simulink library "thermochemical"  (R2017b)
settings: Solver=VariableStepAuto  StartTime=0.0  StopTime=10.0  RelTol=1e-3
values from neighbouring files (symbols this model uses):
  c = conversion_factors()    [blk_clausius_clapeyron.m]    (also in blk_clausius_clapeyron_no_popup.m; blk_cold_room_closed_dry_air.m; blk_reactor_BaCl2_NH3_no_walls.m; blk_reactor_BaCl2_NH3_no_walls_state_space.m)
  cp = metal.cp    [blk_wall_simple.m]    (also in get_metal_properties.m = 390)
  fluid = get_param(blk,'fluid')    [blk_thermodynamic_properties_nonsaturated.m]    (also in blk_thermodynamic_properties_nonsaturated_interpreted.m; blk_thermodynamic_properties_saturated.m; blk_thermodynamic_properties_saturated_interpreted.m; blk_thermodynamic_properties_saturated_mix.m)
  gas = get_material_properties(x.gasName)    [blk_reactor_BaCl2_NH3_cylindrical_no_walls_fun1.m]
  h = get_param(gcb,'ObjectParameters')    [get_param_eval.m]
  rho = metal.rho    [blk_wall_simple.m]    (also in get_metal_properties.m = 8940)
  s = solve(eq,dx,'ReturnConditions',true)    [LMTD_inv.m]    (also in blk_wall_simple.m = get_param_eval(blk,'s'))
  u_gas_at_T_ref = -R * T_ref    [blk_reactor_BaCl2_NH3_no_walls.m]    (also in blk_reactor_BaCl2_NH3_no_walls_state_space.m)
undefined symbols (not defined in the file or in its folder): b_motor, BaCl2, beta, CoolProp, cP_binder, cP_gas, cP_s0, cv, dh_r_0, ENG, heat_exchanger_epsilonNTU_inv_simulink, heat_exchanger_epsilonNTU_simulink, J_motor, K_cin, kappa, Km_motor, La_motor, lookup2D_BreakPoint2, M_binder, N_binder, N_gas_free_volume_init, N_salt, NH3, nh3_v3, nu, P, phase, PID_D_motor, PID_I_motor, PID_P_motor, Ra_motor, Reactor_phase, T, T1, T2, T_init, Tr_init, Tr_ref, U_binder_at_Tr_ref, U_salt_at_X0_Tr_ref, Ur_init, V_void, Valve_regime, Vmax_motor, w_init_motor, X_init
libraries: thermochemical x247, simulink x54, dspsigops x3
(part 9 of 12)

== system thermochemical/Valves/Valve, gas, IEC 60534-2-1:2012 (exact)/Flow computation for compressible fluids, IEC 60534-2-1:2012/Valve regime ==
  In1 : Inport
  In2 : Inport  Port=2
  Enumerated Constant : simulink/Sources/Enumerated Constant  OutDataTypeStr=Enum: Valve_regime  Value=Valve_regime.Open_NonChocked  SampleTime=inf
      settings: SourceProductName=Simulink
  Enumerated Constant1 : simulink/Sources/Enumerated Constant  OutDataTypeStr=Enum: Valve_regime  Value=Valve_regime.Open_Chocked  SampleTime=inf
      settings: SourceProductName=Simulink
  Enumerated Constant2 : simulink/Sources/Enumerated Constant  OutDataTypeStr=Enum: Valve_regime  Value=Valve_regime.Closed  SampleTime=inf
      settings: SourceProductName=Simulink
  Switch1 : Switch  Criteria=u2 > Threshold
  Switch2 : Switch  Criteria=u2 > Threshold  Threshold=1e-5
  Out1 : Outport
  wires:
  In1/1 -> Switch2/2  "valve is closed"
  In2/1 -> Switch1/2  "non-chocked"
  Switch2/1 -> Out1/1  "regime"
  Enumerated Constant2/1 -> Switch2/3  "closed"
  Enumerated Constant1/1 -> Switch1/3  "chocked"
  Enumerated Constant/1 -> Switch1/1  "non-chocked"
  Switch1/1 -> Switch2/1

== system thermochemical/Valves/Valve, gas, IEC 60534-2-1:2012 (modified ideal gas approx.)/Glow computation for compressible fluids, IEC 60534-2-1:2012 (modified ideal gas assumption)/Subsystem ==
  P downstream (bar) : Inport
  P upstream (bar) : Inport  Port=2
  P upstream (bar)1 : Inport  Port=3
  Display{1..5} (5 alike) : Display
  Divide : Product  Inputs=*/
  Divide2 : Product  Inputs=*/
  Gain2 : Gain  Gain=xT
  "Heat capacity ratio of air @ (60°F, 1atm)" : Constant  Value=1.40
  Sign : Signum
  Sum3 : Sum  Inputs=-+
  Sum4 : Sum  Inputs=-+
  Switch1 : Switch  Criteria=u2 > Threshold
  non-chocked : Outport
  non-chocked2 : Outport  Port=2
  non-chocked1 : Outport  Port=3
  wires:
  Divide/1 -> Gain2/1, Display1/1  "Fgamma"
  "Heat capacity ratio of air @ (60°F, 1atm)"/1 -> Divide/2  "gamma air"
  P upstream (bar)1/1 -> Divide/1  "gamma upstream"
  Divide2/1 -> Switch1/1, Sum4/1, Display3/1  "x"
  Sum3/1 -> Divide2/1  "dP"
  Sum4/1 -> Sign/1
  Gain2/1 -> Sum4/2, non-chocked1/1, Display2/1, Switch1/3  "x chocked"
  Sign/1 -> non-chocked/1, Display4/1, Switch1/2  "non-chocked"
  P downstream (bar)/1 -> Sum3/1  "P downstream (bar)"
  P upstream (bar)/1 -> Sum3/2, Divide2/2  "P upstream (bar)"
  Switch1/1 -> non-chocked2/1, Display5/1  "x sizing"

== system thermochemical/Valves/Valve, gas, IEC 60534-2-1:2012 (modified ideal gas approx.)/Glow computation for compressible fluids, IEC 60534-2-1:2012 (modified ideal gas assumption)/Subsystem1 ==
  In1 : Inport
  In2 : Inport  Port=2
  Constant : Constant
  Display4 : Display
  Divide : Product  Inputs=*/
  Gain : Gain  Gain=3
  Sum3 : Sum  Inputs=+-|
  Y : Outport
  wires:
  Constant/1 -> Sum3/1
  In1/1 -> Divide/1  "x sizing"
  Gain/1 -> Divide/2
  Sum3/1 -> Y/1, Display4/1  "Y"
  In2/1 -> Gain/1  "x chocked"
  Divide/1 -> Sum3/2

== system thermochemical/Valves/Valve, gas, IEC 60534-2-1:2012 (modified ideal gas approx.)/Glow computation for compressible fluids, IEC 60534-2-1:2012 (modified ideal gas assumption)/Valve regime ==
  In1 : Inport
  In2 : Inport  Port=2
  Enumerated Constant : simulink/Sources/Enumerated Constant  OutDataTypeStr=Enum: Valve_regime  Value=Valve_regime.Open_NonChocked  SampleTime=inf
      settings: SourceProductName=Simulink
  Enumerated Constant1 : simulink/Sources/Enumerated Constant  OutDataTypeStr=Enum: Valve_regime  Value=Valve_regime.Open_Chocked  SampleTime=inf
      settings: SourceProductName=Simulink
  Enumerated Constant2 : simulink/Sources/Enumerated Constant  OutDataTypeStr=Enum: Valve_regime  Value=Valve_regime.Closed  SampleTime=inf
      settings: SourceProductName=Simulink
  Switch1 : Switch  Criteria=u2 > Threshold
  Switch2 : Switch  Criteria=u2 > Threshold  Threshold=1e-5
  Out1 : Outport
  wires:
  Switch1/1 -> Switch2/1
  Enumerated Constant/1 -> Switch1/1  "non-chocked"
  Enumerated Constant1/1 -> Switch1/3  "chocked"
  Enumerated Constant2/1 -> Switch2/3  "closed"
  Switch2/1 -> Out1/1  "regime"
  In2/1 -> Switch1/2  "non-chocked"
  In1/1 -> Switch2/2  "valve is closed"

== system thermochemical/Valves/Valve, gas, Swagelok model/Gas flow computation ('Swagelok' equations)/Sub-critical (P2 > 1//2 P1) ==
  note: In Matlab script notation:
  note: Reference:
      | Swagelok—TM Swagelok Company
      | © 1994, 1995, 2000, 2002 Swagelok Company
      | December 2007, R4
      | MS-06-84-E
  note: Flow Calculation (in SCFH),
      | sub-critical flow (gas at speed less than the speed of sound)
      | according to 'Swagelok' documentation
  note: % Sub-critical:
      | N2 = 22.67;
      | c = N2 * Pin_psi * (1-2/3*dP_psi/Pin_psi) * sqrt(dP_psi / (Pin_psi*Ggas*Tin_R));
      | SCFM = Cv * c;
      | SCFH = SCFM * 60;
  Ggas : Inport
  Ggas1 : Inport  Port=2
  T1 (°R) : Inport  Port=3
  P1 : Inport  Port=4
  dP : Inport  Port=5
  Constant : Constant
  Divide1 : Product  Inputs=**
  Divide3 : Product  Inputs=/*
  Divide4 : Product  Inputs=/*
  Divide5 : Product  Inputs=***
  Gain5 : Gain  Gain=2/3
  N2 : Gain  Gain=22.67
  Product1 : Product  Inputs=3
  SCFM to SCFH : Gain  Gain=60
  Sqrt : Sqrt  SaturateOnIntegerOverflow=on
  Sum3 : Sum  Inputs=+-|
  c : Outport
  wires:
  dP/1 -> Divide3/2, Divide4/2  "dP (psi)"
  Constant/1 -> Sum3/1
  Ggas/1 -> Product1/1  "Ggas"
  Divide3/1 -> Gain5/1  "dP/P1"
  Gain5/1 -> Sum3/2
  Sqrt/1 -> Divide5/1
  Sum3/1 -> Divide5/3  "1 - 2/3 dP/P1"
  T1 (°R)/1 -> Product1/2  "T1 (°R)"
  Divide5/1 -> N2/1
  Divide4/1 -> Sqrt/1
  N2/1 -> Divide1/2
  Product1/1 -> Divide4/1  "Ggas * T1 * P1"
  P1/1 -> Divide5/2, Product1/3, Divide3/1  "P1 (psi)"
  Ggas1/1 -> Divide1/1  "Cv"
  Divide1/1 -> SCFM to SCFH/1  "SCFM"
  SCFM to SCFH/1 -> c/1  "SCFH"

== system thermochemical/Valves/Valve, gas, Swagelok model/Gas flow computation ('Swagelok' equations)/Super-critical (P2 < 1//2 P1) ==
  note: % Super-critical:
      | N2 = 22.67;
      | c = 0.471 * N2 * Pin_psi * sqrt(1/(Ggas*Tin_R));
      | SCFM = Cv * c;
      | SCFH = SCFM * 60;
  note: Reference:
      | Swagelok—TM Swagelok Company
      | © 1994, 1995, 2000, 2002 Swagelok Company
      | December 2007, R4
      | MS-06-84-E
  note: In Matlab script notation:
  note: Flow Calculation (in SCFH),
      | super-critical (a.k.a. chocked) flow (gas at speed of sound)
      | according to 'Swagelok' documentation
  Ggas : Inport
  Ggas1 : Inport  Port=2
  T1 (°R) : Inport  Port=3
  P1 : Inport  Port=4
  Divide1 : Product  Inputs=**
  Divide5 : Product  Inputs=/*
  N1 : Gain  Gain=0.471
  N2 : Gain  Gain=22.67
  Product1 : Product
  SCFM to SCFH : Gain  Gain=60
  Sqrt : Sqrt  SaturateOnIntegerOverflow=on
  c : Outport
  wires:
  SCFM to SCFH/1 -> c/1  "SCFH"
  Divide1/1 -> SCFM to SCFH/1  "SCFM"
  Ggas1/1 -> Divide1/1  "Cv"
  P1/1 -> Divide5/2  "P1 (psi)"
  Product1/1 -> Sqrt/1  "Ggas * T1"
  N2/1 -> Divide1/2
  Divide5/1 -> N1/1
  T1 (°R)/1 -> Product1/2  "T1 (°R)"
  Sqrt/1 -> Divide5/1
  Ggas/1 -> Product1/1  "Ggas"
  N1/1 -> N2/1

== system thermochemical/Valves/Valve, gas, Swagelok model/Gas flow computation ('Swagelok' equations)/Valve regime ==
  In2 : Inport
  In1 : Inport  Port=2
  Enumerated Constant : simulink/Sources/Enumerated Constant  OutDataTypeStr=Enum: Valve_regime  Value=Valve_regime.Open_NonChocked  SampleTime=inf
      settings: SourceProductName=Simulink
  Enumerated Constant1 : simulink/Sources/Enumerated Constant  OutDataTypeStr=Enum: Valve_regime  Value=Valve_regime.Open_Chocked  SampleTime=inf
      settings: SourceProductName=Simulink
  Enumerated Constant2 : simulink/Sources/Enumerated Constant  OutDataTypeStr=Enum: Valve_regime  Value=Valve_regime.Closed  SampleTime=inf
      settings: SourceProductName=Simulink
  Switch1 : Switch  Criteria=u2 > Threshold
  Switch2 : Switch  Criteria=u2 > Threshold  Threshold=1e-5
  Out1 : Outport
  wires:
  In1/1 -> Switch2/2  "valve is closed"
  In2/1 -> Switch1/2  "P2 - 1/2 P1"
  Switch2/1 -> Out1/1  "regime"
  Enumerated Constant2/1 -> Switch2/3
  Enumerated Constant1/1 -> Switch1/3  "super-critical"
  Enumerated Constant/1 -> Switch1/1  "sub-critical"
  Switch1/1 -> Switch2/1

== system thermochemical/Valves/Valve, liquid (chocked condition not implemented)/Volume flow computation/Turbulent & non-choked flow conditions ==
  note: In Matlab script notation:
  note: Reference:
      | ANSI/ISA-75.01.01 (IEC 60534-2-1 Mod)-2007, eq. 1
  note: Flow Calculation
  note: % GPM computation:
      | N1 = 1;
      | GPM = Cv * N1 * sqrt(dP_psia/SG);
  Ggas : Inport
  dP : Inport  Port=2
  Ggas1 : Inport  Port=3
  Divide1 : Product  Inputs=**
  Divide4 : Product  Inputs=/*
  N1 : Gain
  Sqrt : Sqrt  SaturateOnIntegerOverflow=on
  c : Outport
  wires:
  dP/1 -> Divide4/2  "dP (psi)"
  Ggas/1 -> Divide4/1  "G (dimensionless)"
  Sqrt/1 -> N1/1
  Divide4/1 -> Sqrt/1
  N1/1 -> Divide1/2
  Ggas1/1 -> Divide1/1  "Cv"
  Divide1/1 -> c/1  "US gpm"

== system thermochemical/Valves/Valve, liquid (chocked condition not implemented)/Volume flow computation/Valve regime ==
  In1 : Inport
  Enumerated Constant1 : simulink/Sources/Enumerated Constant  OutDataTypeStr=Enum: Valve_regime  Value=Valve_regime.Open_NonChocked  SampleTime=inf
      settings: SourceProductName=Simulink
  Enumerated Constant2 : simulink/Sources/Enumerated Constant  OutDataTypeStr=Enum: Valve_regime  Value=Valve_regime.Closed  SampleTime=inf
      settings: SourceProductName=Simulink
  Switch2 : Switch  Criteria=u2 > Threshold  Threshold=1e-5
  Out1 : Outport
  wires:
  In1/1 -> Switch2/2  "valve is closed"
  Switch2/1 -> Out1/1  "regime"
  Enumerated Constant2/1 -> Switch2/3
  Enumerated Constant1/1 -> Switch2/1

== system thermochemical/Valves/Valve, liquid, IEC 60534-2-1:2012/Flow computation for incompressible fluids, IEC 60534-2-1:2012/Valve regime ==
  In1 : Inport
  In2 : Inport  Port=2
  Enumerated Constant : simulink/Sources/Enumerated Constant  OutDataTypeStr=Enum: Valve_regime  Value=Valve_regime.Open_NonChocked  SampleTime=inf
      settings: SourceProductName=Simulink
  Enumerated Constant1 : simulink/Sources/Enumerated Constant  OutDataTypeStr=Enum: Valve_regime  Value=Valve_regime.Open_Chocked  SampleTime=inf
      settings: SourceProductName=Simulink
  Enumerated Constant2 : simulink/Sources/Enumerated Constant  OutDataTypeStr=Enum: Valve_regime  Value=Valve_regime.Closed  SampleTime=inf
      settings: SourceProductName=Simulink
  Switch1 : Switch  Criteria=u2 > Threshold
  Switch2 : Switch  Criteria=u2 > Threshold  Threshold=1e-5
  Out1 : Outport
  wires:
  Switch1/1 -> Switch2/1
  Enumerated Constant/1 -> Switch1/1  "non-chocked"
  Enumerated Constant1/1 -> Switch1/3  "chocked"
  Enumerated Constant2/1 -> Switch2/3  "closed"
  Switch2/1 -> Out1/1  "regime"
  In2/1 -> Switch1/2  "non-chocked"
  In1/1 -> Switch2/2  "valve is closed"

== system thermochemical/Valves/Valve, liquid, IEC 60534-2-1:2012/Flow computation for incompressible fluids, IEC 60534-2-1:2012/dP sizing computation ==
  P upstream (bar) : Inport
  P upstream (bar)3 : Inport  Port=2
  P upstream (bar)2 : Inport  Port=3
  P upstream (bar)1 : Inport  Port=4
  Display{1..2,4..5} (4 alike) : Display
  FL factor : Constant  Value=FL
  Sign : Signum
  Sum3 : Sum  Inputs=-+
  Sum4 : Sum  Inputs=|-+
  Switch1 : Switch  Criteria=u2 > Threshold
  dP chocked computation : Subsystem
  non-chocked : Outport
  non-chocked2 : Outport  Port=2
  wires:
  Sum4/1 -> Sign/1
  Sign/1 -> Display4/1, non-chocked/1, Switch1/2  "non-chocked"
  P upstream (bar)/1 -> dP chocked computation/1(P upstream (bar)1), Sum3/2  "P upstream (bar)"
  Switch1/1 -> non-chocked2/1, Display5/1  "dP sizing (bar)"
  P upstream (bar)3/1 -> Sum3/1  "P downstream (bar)"
  Sum3/1 -> Sum4/1, Switch1/1, Display1/1  "dP (bar)"
  dP chocked computation/1(dP chocked (bar)) -> Sum4/2, Switch1/3, Display2/1  "dP chocked (bar)"
  P upstream (bar)2/1 -> dP chocked computation/2(P upstream (bar)2)  "Pv: absolute vapor pressure  of liquid at T upstream (bar)"
  P upstream (bar)1/1 -> dP chocked computation/3(P upstream (bar)3)  "Pc: absolute thermodynamic  critical pressure (bar)"
  FL factor/1 -> dP chocked computation/4(P upstream (bar)4)  "FL factor"

== system thermochemical/Walls/Wall, tube with//without fins/Subsystem1/Subsystem2 ==
  Display{1..4} (4 alike) : Display
  Product2 : Product
  Subsystem : thermochemical/Walls/Wall, tube with//without fins/Subsystem3/Subsystem
      settings: SourceProductName=@ Thermochemical
  Subsystem1 : Subsystem
  Subsystem2 : Subsystem
  Subsystem3 : thermochemical/Walls/Wall, tube with//without fins/Subsystem3/Subsystem3
      settings: SourceProductName=@ Thermochemical
  Switch1 : Switch  Criteria=u2 ~= 0
  s1 : Constant  Value=L_m
  s15 : Constant  Value=pitch_fin_mm
  s18 : Constant  Value=OD_mm
  s19 : Constant  Value=thickness_fin_mm
  s2 : Constant  Value=L_m
  s20 : Constant  Value=height_fin_mm
  s3 : Constant  Value=OD_mm
  s4 : Constant  Value=e_mm
  s5 : Constant  Value=0
  Total tube effective finned area (m2) : Outport
  Inner area (m2) : Outport  Port=2
  wires:
  Switch1/1 -> Display2/1, Total tube effective finned area (m2)/1  "Total finned tube volume (m3)"
  s19/1 -> Subsystem2/2(In2)
  s18/1 -> Subsystem2/1(In1)
  s20/1 -> Subsystem2/3(In4)
  s3/1 -> Subsystem1/1(In1)
  s2/1 -> Subsystem1/3(In3)
  s4/1 -> Subsystem1/2(In2)
  Subsystem1/1(Inner area (m2)) -> Display3/1, Inner area (m2)/1  "Bare tube volume (m3)"
  Subsystem2/1(Inner area (m2)) -> Display4/1, Product2/1
  s1/1 -> Subsystem3/1
  s15/1 -> Subsystem3/2
  Subsystem3/1 -> Display1/1, Product2/2
  Product2/1 -> Switch1/1  "Total finned tube volume (m3)"
  Subsystem/1 -> Switch1/2
  s5/1 -> Switch1/3

== system thermochemical/Walls/Wall, tube with//without fins/Subsystem3/Subsystem ==
  note: Check if any of the fin's parameters is zero
      | (in which case a 'bare tube' is considered)
  Compare To Constant : simulink/Logic and Bit Operations/Compare To Constant  relop=~=  const=0  OutDataTypeStr=boolean
  Mux : Mux  Inputs=3
  Product of Elements : Product  Inputs=*
  s1 : Constant  Value=thickness_fin_mm
  s4 : Constant  Value=pitch_fin_mm
  s5 : Constant  Value=height_fin_mm
  Out1 : Outport
  wires:
  Compare To Constant/1 -> Out1/1  "if == 1 : finned tube if == 0 : bare tube"
  s4/1 -> Mux/3
  s5/1 -> Mux/2
  Product of Elements/1 -> Compare To Constant/1
  s1/1 -> Mux/1
  Mux/1 -> Product of Elements/1

== system thermochemical/Walls/Wall, tube with//without fins/Subsystem3/Subsystem1 ==
  In1 : Inport
  In2 : Inport  Port=2
  In3 : Inport  Port=3
  Gain2 : Gain  Gain=1e-3
  Gain3 : Gain  Gain=1e-3
  Gain5 : Gain  Gain=1e-3
  Gain6 : Gain  Gain=pi
  Product4 : Product
  Sum2 : Sum  Inputs=+-
  Exposed tube area between two fins (m2) : Outport
  wires:
  Gain6/1 -> Product4/2
  Gain2/1 -> Sum2/2
  In2/1 -> Gain2/1  "thickness_fin_mm"
  Gain3/1 -> Gain6/1
  In3/1 -> Gain3/1  "OD_mm"
  In1/1 -> Gain5/1  "pitch_fin_mm"
  Gain5/1 -> Sum2/1
  Sum2/1 -> Product4/1  "Exposed length between two fins (m)"
  Product4/1 -> Exposed tube area between two fins (m2)/1  "Exposed tube area between two fins (m²)"

== system thermochemical/Walls/Wall, tube with//without fins/Subsystem3/Subsystem2 ==
  In1 : Inport
  In2 : Inport  Port=2
  In4 : Inport  Port=3
  Gain1 : Gain  Gain=pi/4
  Gain2 : Gain  Gain=2
  Gain3 : Gain  Gain=1e-3
  Gain4 : Gain  Gain=1e-3
  Gain5 : Gain  Gain=1e-3
  Gain6 : Gain  Gain=pi
  Math Function : Math  Operator=square  SaturateOnIntegerOverflow=on
  Math Function1 : Math  Operator=square  SaturateOnIntegerOverflow=on
  Product1 : Product
  Sum1 : Sum
  Sum2 : Sum  Inputs=+-
  Sum3 : Sum
  Inner area (m2) : Outport
  wires:
  Sum1/1 -> Inner area (m2)/1  "Area of  individual fin (m²)"
  Gain6/1 -> Sum1/2
  Product1/1 -> Gain6/1
  Gain3/1 -> Product1/2  "thickness_fin_m"
  In2/1 -> Gain3/1  "thickness_fin_mm"
  Gain2/1 -> Sum1/1
  Sum3/1 -> Math Function/1, Product1/1
  Gain1/1 -> Gain2/1  "Individual one-side  area of fin (m2)"
  In1/1 -> Gain5/1  "OD_mm"
  In4/1 -> Gain4/1  "height_fin_mm"
  Math Function/1 -> Sum2/1
  Math Function1/1 -> Sum2/2
  Sum2/1 -> Gain1/1
  Gain4/1 -> Sum3/1  "height_fin_m"
  Gain5/1 -> Sum3/2, Math Function1/1  "OD_m"

== system thermochemical/Walls/Wall, tube with//without fins/Subsystem3/Subsystem3 ==
  In1 : Inport
  In2 : Inport  Port=2
  Divide : Product  Inputs=*/
  Gain5 : Gain  Gain=1e-3
  Rounding Function : Rounding
  To avoid 'division by zero' error when pitch is zero : Saturate  UpperLimit=Inf  LowerLimit=1e-7
  Number of fins : Outport
  wires:
  To avoid 'division by zero' error when pitch is zero/1 -> Divide/2
  In2/1 -> Gain5/1  "pitch_fin_mm"
  Gain5/1 -> To avoid 'division by zero' error when pitch is zero/1
  Rounding Function/1 -> Number of fins/1  "Number of fins"
  Divide/1 -> Rounding Function/1
  In1/1 -> Divide/1  "L_m"

== system thermochemical/Walls/Wall, tube with//without fins/Subsystem3/Subsystem4 ==
  In1 : Inport
  In3 : Inport  Port=2
  Gain3 : Gain  Gain=1e-3
  Gain6 : Gain  Gain=pi
  Product4 : Product
  Exposed tube area between two fins (m2) : Outport
  wires:
  Gain6/1 -> Product4/2
  Gain3/1 -> Gain6/1
  Product4/1 -> Exposed tube area between two fins (m2)/1  "Bare tube  external area (m²)"
  In1/1 -> Product4/1  "L_m"
  In3/1 -> Gain3/1  "OD_mm"

== system thermochemical/Walls/Wall, tube with//without fins, with internal heat production/Subsystem1/Subsystem2 ==
  Display{1..4} (4 alike) : Display
  Product2 : Product
  Subsystem : thermochemical/Walls/Wall, tube with//without fins/Subsystem3/Subsystem
      settings: SourceProductName=@ Thermochemical
  Subsystem1 : Subsystem
  Subsystem2 : Subsystem
  Subsystem3 : thermochemical/Walls/Wall, tube with//without fins/Subsystem3/Subsystem3
      settings: SourceProductName=@ Thermochemical
  Switch1 : Switch  Criteria=u2 ~= 0
  s1 : Constant  Value=L_m
  s15 : Constant  Value=pitch_fin_mm
  s18 : Constant  Value=OD_mm
  s19 : Constant  Value=thickness_fin_mm
  s2 : Constant  Value=L_m
  s20 : Constant  Value=height_fin_mm
  s3 : Constant  Value=OD_mm
  s4 : Constant  Value=e_mm
  s5 : Constant  Value=0
  Total tube effective finned area (m2) : Outport
  Inner area (m2) : Outport  Port=2
  wires:
  s5/1 -> Switch1/3
  Subsystem/1 -> Switch1/2
  Product2/1 -> Switch1/1  "Total finned tube volume (m3)"
  Subsystem3/1 -> Product2/2, Display1/1
  s15/1 -> Subsystem3/2
  s1/1 -> Subsystem3/1
  Subsystem2/1(Inner area (m2)) -> Product2/1, Display4/1
  Subsystem1/1(Inner area (m2)) -> Inner area (m2)/1, Display3/1  "Bare tube volume (m3)"
  s4/1 -> Subsystem1/2(In2)
  s2/1 -> Subsystem1/3(In3)
  s3/1 -> Subsystem1/1(In1)
  s20/1 -> Subsystem2/3(In4)
  s18/1 -> Subsystem2/1(In1)
  s19/1 -> Subsystem2/2(In2)
  Switch1/1 -> Total tube effective finned area (m2)/1, Display2/1  "Total finned tube volume (m3)"

== system thermochemical/Walls/Wall, tube with//without fins, with internal heat production/Subsystem3/Subsystem ==
  note: Check if any of the fin's parameters is zero
      | (in which case a 'bare tube' is considered)
  Compare To Constant : simulink/Logic and Bit Operations/Compare To Constant  relop=~=  const=0  OutDataTypeStr=boolean
  Mux : Mux  Inputs=3
  Product of Elements : Product  Inputs=*
  s1 : Constant  Value=thickness_fin_mm
  s4 : Constant  Value=pitch_fin_mm
  s5 : Constant  Value=height_fin_mm
  Out1 : Outport
  wires:
  Mux/1 -> Product of Elements/1
  s1/1 -> Mux/1
  Product of Elements/1 -> Compare To Constant/1
  s5/1 -> Mux/2
  s4/1 -> Mux/3
  Compare To Constant/1 -> Out1/1  "if == 1 : finned tube if == 0 : bare tube"

== system thermochemical/Walls/Wall, tube with//without fins, with internal heat production/Subsystem3/Subsystem1 ==
  In1 : Inport
  In2 : Inport  Port=2
  In3 : Inport  Port=3
  Gain2 : Gain  Gain=1e-3
  Gain3 : Gain  Gain=1e-3
  Gain5 : Gain  Gain=1e-3
  Gain6 : Gain  Gain=pi
  Product4 : Product
  Sum2 : Sum  Inputs=+-
  Exposed tube area between two fins (m2) : Outport
  wires:
  Product4/1 -> Exposed tube area between two fins (m2)/1  "Exposed tube area between two fins (m²)"
  Sum2/1 -> Product4/1  "Exposed length between two fins (m)"
  Gain5/1 -> Sum2/1
  In1/1 -> Gain5/1  "pitch_fin_mm"
  In3/1 -> Gain3/1  "OD_mm"
  Gain3/1 -> Gain6/1
  In2/1 -> Gain2/1  "thickness_fin_mm"
  Gain2/1 -> Sum2/2
  Gain6/1 -> Product4/2

== system thermochemical/Walls/Wall, tube with//without fins, with internal heat production/Subsystem3/Subsystem2 ==
  In1 : Inport
  In2 : Inport  Port=2
  In4 : Inport  Port=3
  Gain1 : Gain  Gain=pi/4
  Gain2 : Gain  Gain=2
  Gain3 : Gain  Gain=1e-3
  Gain4 : Gain  Gain=1e-3
  Gain5 : Gain  Gain=1e-3
  Gain6 : Gain  Gain=pi
  Math Function : Math  Operator=square  SaturateOnIntegerOverflow=on
  Math Function1 : Math  Operator=square  SaturateOnIntegerOverflow=on
  Product1 : Product
  Sum1 : Sum
  Sum2 : Sum  Inputs=+-
  Sum3 : Sum
  Inner area (m2) : Outport
  wires:
  Gain5/1 -> Math Function1/1, Sum3/2  "OD_m"
  Gain4/1 -> Sum3/1  "height_fin_m"
  Sum2/1 -> Gain1/1
  Math Function1/1 -> Sum2/2
  Math Function/1 -> Sum2/1
  In4/1 -> Gain4/1  "height_fin_mm"
  In1/1 -> Gain5/1  "OD_mm"
  Gain1/1 -> Gain2/1  "Individual one-side  area of fin (m2)"
  Sum3/1 -> Product1/1, Math Function/1
  Gain2/1 -> Sum1/1
  In2/1 -> Gain3/1  "thickness_fin_mm"
  Gain3/1 -> Product1/2  "thickness_fin_m"
  Product1/1 -> Gain6/1
  Gain6/1 -> Sum1/2
  Sum1/1 -> Inner area (m2)/1  "Area of  individual fin (m²)"

== system thermochemical/Walls/Wall, tube with//without fins, with internal heat production/Subsystem3/Subsystem3 ==
  In1 : Inport
  In2 : Inport  Port=2
  Divide : Product  Inputs=*/
  Gain5 : Gain  Gain=1e-3
  Rounding Function : Rounding
  To avoid 'division by zero' error when pitch is zero : Saturate  UpperLimit=Inf  LowerLimit=1e-7
  Number of fins : Outport
  wires:
  In1/1 -> Divide/1  "L_m"
  Divide/1 -> Rounding Function/1
  Rounding Function/1 -> Number of fins/1  "Number of fins"
  Gain5/1 -> To avoid 'division by zero' error when pitch is zero/1
  In2/1 -> Gain5/1  "pitch_fin_mm"
  To avoid 'division by zero' error when pitch is zero/1 -> Divide/2

== system thermochemical/Walls/Wall, tube with//without fins, with internal heat production/Subsystem3/Subsystem4 ==
  In1 : Inport
  In3 : Inport  Port=2
  Gain3 : Gain  Gain=1e-3
  Gain6 : Gain  Gain=pi
  Product4 : Product
  Exposed tube area between two fins (m2) : Outport
  wires:
  In3/1 -> Gain3/1  "OD_mm"
  In1/1 -> Product4/1  "L_m"
  Product4/1 -> Exposed tube area between two fins (m2)/1  "Bare tube  external area (m²)"
  Gain3/1 -> Gain6/1
  Gain6/1 -> Product4/2

== system thermochemical/Control volumes/Two-phase saturated fluid control volume (without walls) (without algebraic loop)/Two-phase control volume state-space functions/f1/Subsystem ==
  In2 : Inport
  In3 : Inport  Port=2
  2 : Constant  Value=V
  3 : Constant  Value=V
  Derivative in the two-phase region ∂u/∂v|T : thermochemical/Thermodynamic fluid properties/Derivative in the two-phase region ∂u//∂v|T  fluid=fluid
      settings: SourceProductName=@ Thermochemical
  Product3 : Product  Inputs=**
  Product4 : Product  Inputs=*/
  Product5 : Product  Inputs=*/
  Sum1 : Sum  Inputs=+-
  Terminator : Terminator
  Thermodynamic property (saturated vapor-liquid mix) : thermochemical/Thermodynamic fluid properties/Thermodynamic property  (saturated vapor-liquid mix)  sel=u(T) (J/mol)  fluid=fluid  lookup1D_BreakPoint=0  lookup1D_Data1=fluid.sat.liq.u_molar  lookup1D_Data2=fluid.sat.vap.u_molar
      settings: SourceProductName=@ Thermochemical
  Vapor quality & Liquid volumetric fraction : thermochemical/Thermodynamic fluid properties/Vapor quality & Liquid  volumetric fraction  fluid=fluid
      settings: SourceProductName=@ Thermochemical
  Out1 : Outport
  wires:
  Product4/1 -> Sum1/2
  Sum1/1 -> Product3/1
  Derivative in the two-phase region ∂u/∂v|T/1 -> Sum1/1
  3/1 -> Vapor quality & Liquid volumetric fraction/3
  2/1 -> Product5/1
  Vapor quality & Liquid volumetric fraction/1 -> Thermodynamic property (saturated vapor-liquid mix)/2
  Product3/1 -> Out1/1  "∂U/∂v|T (J.mol/m³) (two-phase)"
  Product5/1 -> Product3/2, Vapor quality & Liquid volumetric fraction/2  "V/v = N (mol)"
  In3/1 -> Product4/2, Product5/2  "v (m3/mol)"
  In2/1 -> Derivative in the two-phase region ∂u/∂v|T/1, Thermodynamic property (saturated vapor-liquid mix)/1, Vapor quality & Liquid volumetric fraction/1  "T (K)"
  Thermodynamic property (saturated vapor-liquid mix)/1 -> Product4/1
  Vapor quality & Liquid volumetric fraction/2 -> Terminator/1

== system thermochemical/Control volumes/Two-phase saturated fluid control volume (without walls) (without algebraic loop)/Two-phase control volume state-space functions/f1/Subsystem1 ==
  In2 : Inport
  In3 : Inport  Port=2
  2 : Constant  Value=V
  3 : Constant  Value=V
  Derivative in the two-phase region ∂u/∂T|v : thermochemical/Thermodynamic fluid properties/Derivative in the two-phase region ∂u//∂T|v  fluid=fluid
      settings: SourceProductName=@ Thermochemical
  Product3 : Product  Inputs=**
  Product5 : Product  Inputs=*/
  Terminator : Terminator
  Vapor quality & Liquid volumetric fraction : thermochemical/Thermodynamic fluid properties/Vapor quality & Liquid  volumetric fraction  fluid=fluid
      settings: SourceProductName=@ Thermochemical
  Out1 : Outport
  wires:
  Vapor quality & Liquid volumetric fraction/2 -> Terminator/1
  In2/1 -> Derivative in the two-phase region ∂u/∂T|v/1, Vapor quality & Liquid volumetric fraction/1  "T (K)"
  In3/1 -> Product5/2  "v (m3/mol)"
  Product5/1 -> Product3/2, Vapor quality & Liquid volumetric fraction/2  "V/v = N (mol)"
  Product3/1 -> Out1/1  "∂U/∂T|v (J/K) (two-phase)"
  Vapor quality & Liquid volumetric fraction/1 -> Derivative in the two-phase region ∂u/∂T|v/2
  2/1 -> Product5/1
  3/1 -> Vapor quality & Liquid volumetric fraction/3
  Derivative in the two-phase region ∂u/∂T|v/1 -> Product3/1

== system thermochemical/Heat exchangers/Heat Exchanger, e-NTU method (UA input) Loop 2: water/Subsystem/Subsystem1/Average ==
  In1 : Inport
  In2 : Inport  Port=2
  Gain : Gain  Gain=0.5
  Sum : Sum
  Out1 : Outport
  wires:
  Gain/1 -> Out1/1  "avg"
  In1/1 -> Sum/1  "In 1"
  In2/1 -> Sum/2  "In 2"
  Sum/1 -> Gain/1

== system thermochemical/Heat exchangers/Heat Exchanger, e-NTU method (epsilon input) Loop 2: water/Subsystem/Subsystem1/Average ==
  In1 : Inport
  In2 : Inport  Port=2
  Gain : Gain  Gain=0.5
  Sum : Sum
  Out1 : Outport
  wires:
  Sum/1 -> Gain/1
  In2/1 -> Sum/2  "In 2"
  In1/1 -> Sum/1  "In 1"
  Gain/1 -> Out1/1  "avg"

== system thermochemical/Reactors/Reactor, BaCl2//NH3, state-space form, [Tr, Ng, X] as state variables, no algebraic loops, ideal gas in void volume, ideal gas in salt/Reactor, BaCl2//NH3, no walls, state-space form, [Tr, Ng, X] as state variables, no algebraic loops, ideal gas in void volume/Reactor, no walls, state space form/Reactor output function ==
  In1 : Inport
  Clausius-Clapeyron : thermochemical/Thermodynamic fluid properties/Clausius-Clapeyron  sel_1=P(T)  sel_2=BaCl2/NH3
      settings: SourceProductName=@ Thermochemical
  Demux : Demux  Outputs=3
  Enthalpy of ideal gas : thermochemical/Thermodynamic fluid properties/Enthalpy of ideal gas  T_ref=T_ref  cP_gas=cP_gas  h_gas_at_T_ref="u_gas_at_T_ref  + R * T_ref"
      settings: SourceProductName=@ Thermochemical
  Gain4 : Gain  Gain=nu*N_salt
  Gain7 : Gain  Gain=1/V_void
  Ideal gas equation of state : thermochemical/Thermodynamic fluid properties/Ideal gas equation of state  sel=P(T,rho)  R=8.3145  Pa_to_bar=1e-5  bar_to_Pa=1e5
      settings: SourceProductName=@ Thermochemical
  Mux : Mux
  Reactor phase : Subsystem
  Reactor's internal energy equation : thermochemical/Reactors/Reactor's internal energy equation  Tr_ref=T_ref  N_salt=N_salt  cP_s0=cP_s0  U_salt_at_X0_Tr_ref=U_salt_at_X0_T_ref  N_binder=N_binder  M_binder=M_binder  cP_binder=cP_binder  U_binder_at_Tr_ref=U_binder_at_T_ref  V_void=V_void  gas_model_void_volume=Ideal gas model  gas_model_salt=Ideal gas model  is_ideal_gas_in_void_volume=1  is_ideal_gas_in_salt=1  fluid=fluid  cP_gas=cP_gas  u_gas_at_Tr_ref=u_gas_at_T_ref  nu=nu  dh_r=dh_r_0  R=8.314472
      settings: SourceProductName=@ Thermochemical
  Sum16 : Sum  Inputs=+-|
  Sum4 : Sum  Inputs=|+-
  Terminator : Terminator
  Out1 : Outport
  Out2 : Outport  Port=2
  wires:
  Demux/3 -> Gain4/1, Mux/3, Reactor's internal energy equation/1  "x(3) = X (0..1)"
  Demux/1 -> Mux/1, Clausius-Clapeyron/1, Enthalpy of ideal gas/1, Ideal gas equation of state/1, Reactor's internal energy equation/3  "x(1) = T (K)"
  Reactor's internal energy equation/1 -> Terminator/1  "Ur (J)"
  Demux/2 -> Sum4/1  "x(2) = Ngas,total (mol)"
  Sum16/1 -> Reactor phase/1(In1)
  Clausius-Clapeyron/1 -> Sum16/2  "P eq (bar)"
  Reactor phase/1(Out1) -> Out2/1  "Reactor phase"
  Gain7/1 -> Ideal gas equation of state/2
  Enthalpy of ideal gas/1 -> Mux/4  "h gas free volume (J/mol)"
  Ideal gas equation of state/1 -> Mux/2, Sum16/1  "P (bar)"
  Sum4/1 -> Reactor's internal energy equation/2, Gain7/1  "Ngas,void"
  Gain4/1 -> Sum4/2
  Mux/1 -> Out1/1  "Y(vector)"
  In1/1 -> Demux/1  "X(vector)"

== system thermochemical/Reactors/Reactor, BaCl2//NH3, state-space form, [Tr, Ng, X] as state variables, no algebraic loops, ideal gas in void volume, ideal gas in salt/Reactor, BaCl2//NH3, no walls, state-space form, [Tr, Ng, X] as state variables, no algebraic loops, ideal gas in void volume/Reactor, no walls, state space form/Reactor state-space functions ==
  In1 : Inport
  In2 : Inport  Port=2
  Mux : Mux  Inputs=3
  f1 : Subsystem
  f2 : Subsystem
  f3 : Subsystem
  Out2 : Outport
  wires:
  In2/1 -> f1/2(In1), f3/2(In2), f2/2(In2)  "U(vector)"
  In1/1 -> f1/1(In6), f2/1(In6), f3/1(In6)  "X(vector)"
  Mux/1 -> Out2/1  "dX/dt(vector)"
  f1/1(Out2) -> Mux/1
  f3/1(Out2) -> Mux/3
  f2/1(Out2) -> Mux/2

== system thermochemical/Reactors/Reactor, BaCl2//NH3, state-space form, [Tr, Ng, X] as state variables, no algebraic loops, real gas in void volume, ideal gas in salt/Reactor, BaCl2//NH3, no walls, state-space form, [Tr, Ng, X] as state variables, no algebraic loops, real gas in void volume, ideal gas in salt/Reactor, no walls, state space form/Reactor output function ==
  In1 : Inport
  Clausius-Clapeyron : thermochemical/Thermodynamic fluid properties/Clausius-Clapeyron  sel_1=P(T)  sel_2=BaCl2/NH3
      settings: SourceProductName=@ Thermochemical
  Demux : Demux  Outputs=3
  Gain4 : Gain  Gain=nu*N_salt
  Gain7 : Gain  Gain=1/V_void
  Mux : Mux
  Reactor phase : Subsystem
  Reactor's internal energy equation : thermochemical/Reactors/Reactor's internal energy equation  Tr_ref=T_ref  N_salt=N_salt  cP_s0=cP_s0  U_salt_at_X0_Tr_ref=U_salt_at_X0_T_ref  N_binder=N_binder  M_binder=M_binder  cP_binder=cP_binder  U_binder_at_Tr_ref=U_binder_at_T_ref  V_void=V_void  gas_model_void_volume=Real gas model  gas_model_salt=Ideal gas model  is_ideal_gas_in_void_volume=-1  is_ideal_gas_in_salt=1  fluid=fluid  cP_gas=cP_gas  u_gas_at_Tr_ref=u_gas_at_T_ref  nu=nu  dh_r=dh_r_0  R=8.314472
      settings: SourceProductName=@ Thermochemical
  Sum16 : Sum  Inputs=+-|
  Sum4 : Sum  Inputs=|+-
  Terminator : Terminator
  Thermodynamic property (non-saturated) : thermochemical/Thermodynamic fluid properties/Thermodynamic  property (non-saturated)  sel=h(T,rho)  fluid=fluid  reciprocVar=-1  lookup2D_BreakPoint1=fluid.no_sat.T_rho_indep.var_indep.T  lookup2D_BreakPoint2=fluid.no_sat.T_rho_indep.var_indep.rho_molar  lookup2D_Data=fluid.no_sat.T_rho_indep.var_dep.h_molar
      settings: SourceProductName=@ Thermochemical
  Thermodynamic property (non-saturated)1 : thermochemical/Thermodynamic fluid properties/Thermodynamic  property (non-saturated)  sel=P(T,rho)  fluid=fluid  reciprocVar=-1  lookup2D_BreakPoint1=fluid.no_sat.T_rho_indep.var_indep.T  lookup2D_BreakPoint2=fluid.no_sat.T_rho_indep.var_indep.rho_molar  lookup2D_Data=fluid.no_sat.T_rho_indep.var_dep.P
      settings: SourceProductName=@ Thermochemical
  Out1 : Outport
  Out2 : Outport  Port=2
  wires:
  Reactor's internal energy equation/1 -> Terminator/1  "Ur (J)"
  In1/1 -> Demux/1  "X(vector)"
  Mux/1 -> Out1/1  "Y(vector)"
  Gain4/1 -> Sum4/2
  Sum4/1 -> Reactor's internal energy equation/2, Gain7/1  "Ngas,void"
  Thermodynamic property (non-saturated)1/1 -> Sum16/1, Mux/2  "P (bar)"
  Demux/3 -> Mux/3, Gain4/1, Reactor's internal energy equation/1  "X (0..1)"
  Thermodynamic property (non-saturated)/1 -> Mux/4  "h gas free volume (J/mol)"
  Demux/2 -> Sum4/1  "Ngas,total (mol)"
  Demux/1 -> Clausius-Clapeyron/1, Thermodynamic property (non-saturated)/1, Thermodynamic property (non-saturated)1/1, Mux/1, Reactor's internal energy equation/3  "T (K)"
  Gain7/1 -> Thermodynamic property (non-saturated)/2, Thermodynamic property (non-saturated)1/2
  Reactor phase/1(Out1) -> Out2/1  "Reactor phase"
  Clausius-Clapeyron/1 -> Sum16/2  "P eq (bar)"
  Sum16/1 -> Reactor phase/1(In1)

== system thermochemical/Reactors/Reactor, BaCl2//NH3, state-space form, [Tr, Ng, X] as state variables, no algebraic loops, real gas in void volume, ideal gas in salt/Reactor, BaCl2//NH3, no walls, state-space form, [Tr, Ng, X] as state variables, no algebraic loops, real gas in void volume, ideal gas in salt/Reactor, no walls, state space form/Reactor state-space functions ==
  In1 : Inport
  In2 : Inport  Port=2
  Mux : Mux  Inputs=3
  f1 : Subsystem
  f2 : Subsystem
  f3 : Subsystem
  Out2 : Outport
  wires:
  f2/1(Out2) -> Mux/2
  f3/1(Out2) -> Mux/3
  f1/1(Out2) -> Mux/1
  Mux/1 -> Out2/1  "dX/dt(vector)"
  In1/1 -> f3/1(In6), f2/1(In6), f1/1(In6)  "X(vector)"
  In2/1 -> f2/2(In2), f3/2(In2), f1/2(In1)  "U(vector)"

== system thermochemical/Reactors/Reactor, BaCl2//NH3, state-space form, [Tr, Ng, X] as state variables, no algebraic loops, real gas in void volume, real gas in salt/Reactor, BaCl2//NH3, no walls, state-space form, [Tr, Ng, X] as state variables, no algebraic loops, real gas in void volume, real gas in salt/Reactor, no walls, state space form/Reactor output function ==
  In1 : Inport
  Clausius-Clapeyron : thermochemical/Thermodynamic fluid properties/Clausius-Clapeyron  sel_1=P(T)  sel_2=BaCl2/NH3
      settings: SourceProductName=@ Thermochemical
  Demux : Demux  Outputs=3
  Gain4 : Gain  Gain=nu*N_salt
  Gain7 : Gain  Gain=1/V_void
  Mux : Mux
  Reactor phase : Subsystem
  Reactor's internal energy equation : thermochemical/Reactors/Reactor's internal energy equation  Tr_ref=T_ref  N_salt=N_salt  cP_s0=cP_s0  U_salt_at_X0_Tr_ref=U_salt_at_X0_T_ref  N_binder=N_binder  M_binder=M_binder  cP_binder=cP_binder  U_binder_at_Tr_ref=U_binder_at_T_ref  V_void=V_void  gas_model_void_volume=Real gas model  gas_model_salt=Real gas model  is_ideal_gas_in_void_volume=-1  is_ideal_gas_in_salt=-1  fluid=fluid  cP_gas=cP_gas  u_gas_at_Tr_ref=u_gas_at_T_ref  nu=nu  dh_r=dh_r_0  R=8.314472
      settings: SourceProductName=@ Thermochemical
  Sum16 : Sum  Inputs=+-|
  Sum4 : Sum  Inputs=|+-
  Terminator : Terminator
  Thermodynamic property (non-saturated) : thermochemical/Thermodynamic fluid properties/Thermodynamic  property (non-saturated)  sel=h(T,rho)  fluid=fluid  reciprocVar=-1  lookup2D_BreakPoint1=fluid.no_sat.T_rho_indep.var_indep.T  lookup2D_BreakPoint2=fluid.no_sat.T_rho_indep.var_indep.rho_molar  lookup2D_Data=fluid.no_sat.T_rho_indep.var_dep.h_molar
      settings: SourceProductName=@ Thermochemical
  Thermodynamic property (non-saturated)1 : thermochemical/Thermodynamic fluid properties/Thermodynamic  property (non-saturated)  sel=P(T,rho)  fluid=fluid  reciprocVar=-1  lookup2D_BreakPoint1=fluid.no_sat.T_rho_indep.var_indep.T  lookup2D_BreakPoint2=fluid.no_sat.T_rho_indep.var_indep.rho_molar  lookup2D_Data=fluid.no_sat.T_rho_indep.var_dep.P
      settings: SourceProductName=@ Thermochemical
  Out1 : Outport
  Out2 : Outport  Port=2
  wires:
  Sum16/1 -> Reactor phase/1(In1)
  Clausius-Clapeyron/1 -> Sum16/2  "P eq (bar)"
  Reactor phase/1(Out1) -> Out2/1  "Reactor phase"
  Gain7/1 -> Thermodynamic property (non-saturated)1/2, Thermodynamic property (non-saturated)/2
  Demux/1 -> Reactor's internal energy equation/3, Mux/1, Thermodynamic property (non-saturated)1/1, Thermodynamic property (non-saturated)/1, Clausius-Clapeyron/1  "T (K)"
  Demux/2 -> Sum4/1  "Ngas,total (mol)"
  Thermodynamic property (non-saturated)/1 -> Mux/4  "h gas free volume (J/mol)"
  Demux/3 -> Reactor's internal energy equation/1, Gain4/1, Mux/3  "X (0..1)"
  Thermodynamic property (non-saturated)1/1 -> Mux/2, Sum16/1  "P (bar)"
  Sum4/1 -> Reactor's internal energy equation/2, Gain7/1  "Ngas,void"
  Gain4/1 -> Sum4/2
  Mux/1 -> Out1/1  "Y(vector)"
  In1/1 -> Demux/1  "X(vector)"
  Reactor's internal energy equation/1 -> Terminator/1  "Ur (J)"

== system thermochemical/Reactors/Reactor, BaCl2//NH3, state-space form, [Tr, Ng, X] as state variables, no algebraic loops, real gas in void volume, real gas in salt/Reactor, BaCl2//NH3, no walls, state-space form, [Tr, Ng, X] as state variables, no algebraic loops, real gas in void volume, real gas in salt/Reactor, no walls, state space form/Reactor state-space functions ==
  In1 : Inport
  In2 : Inport  Port=2
  Mux : Mux  Inputs=3
  f1 : Subsystem
  f2 : Subsystem
  f3 : Subsystem
  Out2 : Outport
  wires:
  In2/1 -> f1/2(In1), f3/2(In2), f2/2(In2)  "U(vector)"
  In1/1 -> f1/1(In6), f2/1(In6), f3/1(In6)  "X(vector)"
  Mux/1 -> Out2/1  "dX/dt(vector)"
  f1/1(Out2) -> Mux/1
  f3/1(Out2) -> Mux/3
  f2/1(Out2) -> Mux/2

== system thermochemical/Reactors/Reactor, BaCl2//NH3, state-space form, [Ur, Ng, X] as state variables, no algebraic loops, ideal gas in void volume, ideal gas in salt/Reactor, BaCl2//NH3, no walls, state-space form, [Ur, Ng, X] as state variables, no algebraic loops, ideal gas in void volume, ideal gas in salt/Reactor, no walls, state space form/Initial conditions ==
  Gain1 : Gain  Gain=N_salt * nu
  Initial condition : Constant  Value=X_init
  Initial condition1 : Constant  Value=N_gas_free_volume_init
  Initial condition2 : Constant  Value=Tr_init
  Mux : Mux  Inputs=3
  Reactor's internal energy equation : thermochemical/Reactors/Reactor's internal energy equation  Tr_ref=T_ref  N_salt=N_salt  cP_s0=cP_s0  U_salt_at_X0_Tr_ref=U_salt_at_X0_T_ref  N_binder=N_binder  M_binder=M_binder  cP_binder=cP_binder  U_binder_at_Tr_ref=U_binder_at_T_ref  V_void=V_void  gas_model_void_volume=Ideal gas model  gas_model_salt=Ideal gas model  is_ideal_gas_in_void_volume=1  is_ideal_gas_in_salt=1  fluid=fluid  cP_gas=cP_gas  u_gas_at_Tr_ref=u_gas_at_T_ref  nu=nu  dh_r=dh_r_0  R=8.314472
      settings: SourceProductName=@ Thermochemical
  Sum4 : Sum  Inputs=++|
  Out2 : Outport
  wires:
  Mux/1 -> Out2/1  "X0 (vector)"
  Initial condition/1 -> Reactor's internal energy equation/1, Gain1/1, Mux/3  "x(3) = X (0..1)"
  Initial condition1/1 -> Reactor's internal energy equation/2, Sum4/1
  Reactor's internal energy equation/1 -> Mux/1  "x(1) = Ur (J)"
  Initial condition2/1 -> Reactor's internal energy equation/3
  Sum4/1 -> Mux/2  "x(2) = Ngas,total (mol)"
  Gain1/1 -> Sum4/2

== system thermochemical/Reactors/Reactor, BaCl2//NH3, state-space form, [Ur, Ng, X] as state variables, no algebraic loops, ideal gas in void volume, ideal gas in salt/Reactor, BaCl2//NH3, no walls, state-space form, [Ur, Ng, X] as state variables, no algebraic loops, ideal gas in void volume, ideal gas in salt/Reactor, no walls, state space form/Reactor output function ==
  In1 : Inport
  Clausius-Clapeyron : thermochemical/Thermodynamic fluid properties/Clausius-Clapeyron  sel_1=P(T)  sel_2=BaCl2/NH3
      settings: SourceProductName=@ Thermochemical
  Demux : Demux  Outputs=3
  Enthalpy of ideal gas : thermochemical/Thermodynamic fluid properties/Enthalpy of ideal gas  T_ref=T_ref  cP_gas=cP_gas  h_gas_at_T_ref="u_gas_at_T_ref  + R * T_ref"
      settings: SourceProductName=@ Thermochemical
  Gain4 : Gain  Gain=nu*N_salt
  Gain7 : Gain  Gain=1/V_void
  Ideal gas equation of state : thermochemical/Thermodynamic fluid properties/Ideal gas equation of state  sel=P(T,rho)  R=8.3145  Pa_to_bar=1e-5  bar_to_Pa=1e5
      settings: SourceProductName=@ Thermochemical
  Mux : Mux
  Reactor phase : Subsystem
  Sum16 : Sum  Inputs=+-|
  Sum4 : Sum  Inputs=|+-
  Tr = inv(g[X(vector)]) : thermochemical/Reactors/Reactor, BaCl2//NH3, state-space form, [Ur, Ng, X] as state variables, no algebraic loops, ideal gas in void volume, ideal gas in salt/Reactor, BaCl2//NH3, no walls, state-space form, [Ur, Ng, X] as state variables, no algebraic loops, ideal gas in void volume, ideal gas in salt/Reactor, no walls, state space form/Reactor state-space functions/f1/Tr = inv(g[X(vector)])
      settings: SourceProductName=@ Thermochemical
  Out1 : Outport
  Out2 : Outport  Port=2
  wires:
  Sum16/1 -> Reactor phase/1(In1)
  Clausius-Clapeyron/1 -> Sum16/2  "P eq (bar)"
  Reactor phase/1(Out1) -> Out2/1  "Reactor phase"
  Gain7/1 -> Ideal gas equation of state/2
  Tr = inv(g[X(vector)])/1 -> Clausius-Clapeyron/1, Enthalpy of ideal gas/1, Ideal gas equation of state/1, Mux/1  "Tr (K)"
  Demux/2 -> Tr = inv(g[X(vector)])/2, Sum4/1  "Ngas,total (mol)"
  Enthalpy of ideal gas/1 -> Mux/4  "h gas free volume (J/mol)"
  Demux/3 -> Tr = inv(g[X(vector)])/3, Mux/3, Gain4/1  "X (0..1)"
  Ideal gas equation of state/1 -> Sum16/1, Mux/2  "P (bar)"
  Sum4/1 -> Gain7/1  "Ngas,void"
  Gain4/1 -> Sum4/2
  Mux/1 -> Out1/1  "Y(vector)"
  In1/1 -> Demux/1  "X(vector)"
  Demux/1 -> Tr = inv(g[X(vector)])/1  "Ur (J)"

== system thermochemical/Reactors/Reactor, BaCl2//NH3, state-space form, [Ur, Ng, X] as state variables, no algebraic loops, ideal gas in void volume, ideal gas in salt/Reactor, BaCl2//NH3, no walls, state-space form, [Ur, Ng, X] as state variables, no algebraic loops, ideal gas in void volume, ideal gas in salt/Reactor, no walls, state space form/Reactor state-space functions ==
  In1 : Inport
  In2 : Inport  Port=2
  Mux : Mux  Inputs=3
  f1 : Subsystem
  f2 : Subsystem
  f3 : Subsystem
  Out2 : Outport
  wires:
  In2/1 -> f1/2(In2), f3/2(In2), f2/2(In2)  "U (vector)"
  In1/1 -> f1/1(In6), f2/1(In6), f3/1(In6)  "X (vector)"
  Mux/1 -> Out2/1  "dX/dt (vector)"
  f1/1(Out2) -> Mux/1
  f3/1(Out2) -> Mux/3
  f2/1(Out2) -> Mux/2

== system thermochemical/Reactors/Reactor, BaCl2//NH3, with algebraic loops, ideal gas in void volume, ideal gas in salt/Reactor, BaCl2//NH3, no walls, with algebraic loops, ideal gas in void volume, ideal gas in salt/Reactor (no walls)/Reactor's internal energy differential equation ==
  note: Reactor - Internal energy's
      | differential equation
  In1 : Inport
  In2 : Inport  Port=2
  In5 : Inport  Port=3
  In3 : Inport  Port=4
  1 : Constant  Value=X_init
  2 : Constant  Value=N_gas_free_volume_init
  3 : Constant  Value=Tr_init
  Integrator6 : Integrator  InitialConditionSource=external  InitialCondition=Ur_init
  Product4 : Product
  Reactor's internal energy equation : thermochemical/Reactors/Reactor's internal energy equation  Tr_ref=T_ref  N_salt=N_salt  cP_s0=cP_s0  U_salt_at_X0_Tr_ref=U_salt_at_X0_T_ref  N_binder=N_binder  M_binder=M_binder  cP_binder=cP_binder  U_binder_at_Tr_ref=U_binder_at_T_ref  V_void=V_void  gas_model_void_volume=Ideal gas model  gas_model_salt=Ideal gas model  is_ideal_gas_in_void_volume=1  is_ideal_gas_in_salt=1  fluid=fluid  cP_gas=cP_gas  u_gas_at_Tr_ref=u_gas_at_T_ref  nu=nu  dh_r=dh_r_0  R=8.314472
      settings: SourceProductName=@ Thermochemical
  Relay : Relay  OnSwitchValue=dn_dead_zone  OffSwitchValue=-dn_dead_zone  OffOutputValue=-1
  Sum19 : Sum  Inputs=++|
  Switch1 : Switch
  Out1 : Outport
  wires:
  In3/1 -> Relay/1, Product4/2  "dn_gas (mol/sec) > 0: gas in   < 0: gas out"
  In5/1 -> Switch1/3  "enthalpy out (J/mol)"
  In1/1 -> Sum19/1  "q out → in (W)"
  Sum19/1 -> Integrator6/1  "dUr"
  Integrator6/1 -> Out1/1  "U_reactor (J)"
  In2/1 -> Switch1/1  "enthalpy in (J/mol)"
  Switch1/1 -> Product4/1  "h_gas(Tgas)"
  Product4/1 -> Sum19/2  "dn_gas * h_gas"
  Reactor's internal energy equation/1 -> Integrator6/2
  1/1 -> Reactor's internal energy equation/1
  3/1 -> Reactor's internal energy equation/3
  2/1 -> Reactor's internal energy equation/2
  Relay/1 -> Switch1/2

== system thermochemical/Reactors/Reactor, BaCl2//NH3, with algebraic loops, ideal gas in void volume, ideal gas in salt/Reactor, BaCl2//NH3, no walls, with algebraic loops, ideal gas in void volume, ideal gas in salt/Reactor (no walls)/Reactor's temperature and pressure ==
  In2 : Inport
  In1 : Inport  Port=2
  "Reaction kinetic, differential equation" : Subsystem
  Reactor's energy balance : Subsystem
  Out3 : Outport
  Out1 : Outport  Port=2
  Out2 : Outport  Port=3
  Out4 : Outport  Port=4
  wires:
  In1/1 -> Reactor's energy balance/1(In1)  "U_reactor (J)"
  "Reaction kinetic, differential equation"/2(Out2) -> Out4/1, Reactor's energy balance/3(In3)  "X (0..1)"
  Reactor's energy balance/1(Out1) -> "Reaction kinetic, differential equation"/1(In1), Out3/1  "T_reactor (K)"
  In2/1 -> Reactor's energy balance/2(In2)  "N_gas_reactor (mol)"
  Reactor's energy balance/2(Out2) -> "Reaction kinetic, differential equation"/2(In2), Out1/1  "P_reactor (bar)"
  "Reaction kinetic, differential equation"/1(Out1) -> Out2/1  "Reactor phase"

== system thermochemical/Reactors/Reactor, BaCl2//NH3, with algebraic loops, real gas in void volume, ideal gas in salt/Reactor, BaCl2//NH3, no walls, with algebraic loops, real gas in void volume, ideal gas in salt/Reactor (no walls)/Reactor's internal energy differential equation ==
  note: Reactor - Internal energy's
      | differential equation
  In1 : Inport
  In2 : Inport  Port=2
  In5 : Inport  Port=3
  In3 : Inport  Port=4
  1 : Constant  Value=X_init
  2 : Constant  Value=N_gas_free_volume_init
  3 : Constant  Value=Tr_init
  Integrator6 : Integrator  InitialConditionSource=external  InitialCondition=Ur_init
  Product4 : Product
  Reactor's internal energy equation : thermochemical/Reactors/Reactor's internal energy equation  Tr_ref=T_ref  N_salt=N_salt  cP_s0=cP_s0  U_salt_at_X0_Tr_ref=U_salt_at_X0_T_ref  N_binder=N_binder  M_binder=M_binder  cP_binder=cP_binder  U_binder_at_Tr_ref=U_binder_at_T_ref  V_void=V_void  gas_model_void_volume=Real gas model  gas_model_salt=Ideal gas model  is_ideal_gas_in_void_volume=-1  is_ideal_gas_in_salt=1  fluid=fluid  cP_gas=cP_gas  u_gas_at_Tr_ref=u_gas_at_T_ref  nu=nu  dh_r=dh_r_0  R=8.314472
      settings: SourceProductName=@ Thermochemical
  Relay : Relay  OnSwitchValue=dn_dead_zone  OffSwitchValue=-dn_dead_zone  OffOutputValue=-1
  Sum19 : Sum  Inputs=++|
  Switch1 : Switch
  Out1 : Outport
  wires:
  Relay/1 -> Switch1/2
  2/1 -> Reactor's internal energy equation/2
  3/1 -> Reactor's internal energy equation/3
  1/1 -> Reactor's internal energy equation/1
  Reactor's internal energy equation/1 -> Integrator6/2
  Product4/1 -> Sum19/2  "dn_gas * h_gas"
  Switch1/1 -> Product4/1  "h_gas(Tgas)"
  In2/1 -> Switch1/1  "enthalpy in (J/mol)"
  Integrator6/1 -> Out1/1  "U_reactor (J)"
  Sum19/1 -> Integrator6/1  "dUr"
  In1/1 -> Sum19/1  "q out → in (W)"
  In5/1 -> Switch1/3  "enthalpy out (J/mol)"
  In3/1 -> Product4/2, Relay/1  "dn_gas (mol/sec) > 0: gas in   < 0: gas out"
